simulink model "EngModelJumpRamp"  (R2013a)
settings: Solver=ode15s  StartTime=0.0  StopTime=10.0  RelTol=1e-5
values from neighbouring files (symbols this model uses):
  AFlowcontrol = AFhighc    (= 23)    [init_ele.m]
  AFn = 27*ones(engines,1)    [initHybrid.m]    (also in initMV.m; init_ele.m = 27)
  ma0 = .2*ones(engines,1)    [initHybrid.m]    (also in initMV.m; init_ele.m = 0.2)
  nr = 1    [init_ele.m]
undefined symbols (not defined in the file or in its folder): Kappa1, magnitude, pin0
undefined symbols (not defined in the file): generators
libraries: simulink x2, EngineSystemSubmodel x1
settings Model: Creator=yum  LastModifiedBy=yum
settings DebuggingCC: SolverPrmCheckMsg=none

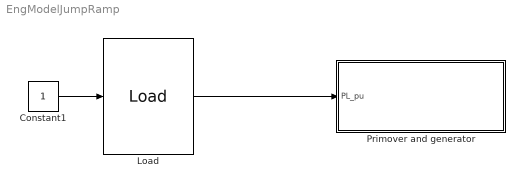
== system EngModelJumpRamp ==
  Constant1 : Constant
  Load : EngineSystemSubmodel/Load  Load_index=Load_index  Load_amp=Load_amp  Load_bias=Load_bias  Start_time=Start_time  T_load=T_load
  Primover and generator : Subsystem  mask{genset=generators(1)}
      mask prompts: genset "Genset parameters"
  wires:
  Load/1 -> Primover and generator/1(PL_pu)
  Constant1/1 -> Load/1

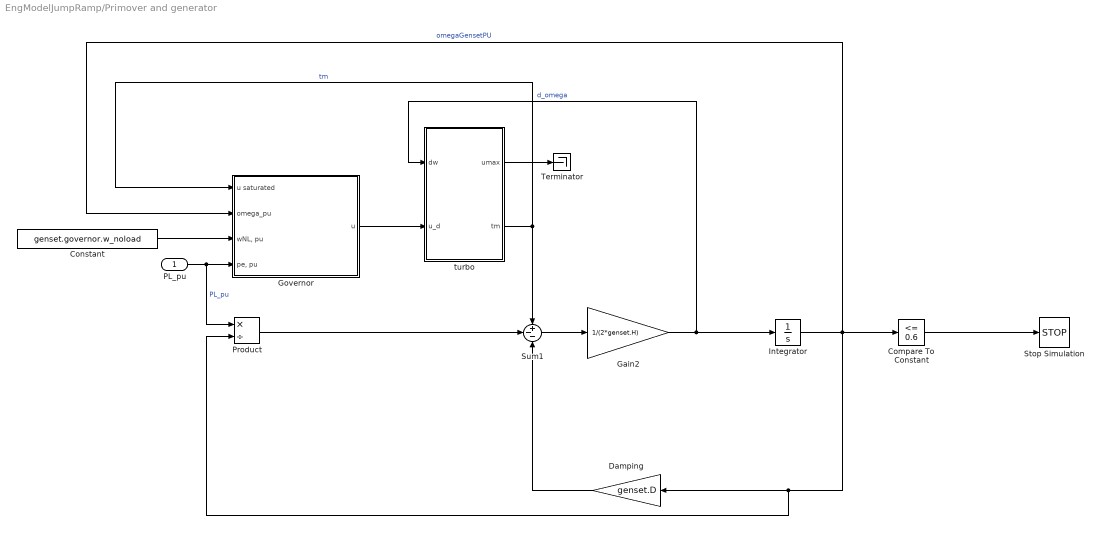
== system EngModelJumpRamp/Primover and generator ==
  PL_pu : Inport
  Compare To Constant : simulink/Logic and Bit Operations/Compare To Constant  relop=<=  const=0.6  OutDataTypeStr=boolean
  Constant : Constant  Value=genset.governor.w_noload
  Damping : Gain  Gain=genset.D
  Gain2 : Gain  Gain=1/(2*genset.H)
  Governor : Subsystem
  Integrator : Integrator  InitialCondition=genset.omega0
  Product : Product  Inputs=*/
  Stop Simulation : Stop
  Sum1 : Sum  Inputs=+--
  Terminator : Terminator
  turbo : Subsystem
  wires:
  Governor/1(u) -> turbo/2(u_d)
  turbo/2(tm) -> Sum1/1, Governor/1(u saturated)  "tm"
  Sum1/1 -> Gain2/1
  Gain2/1 -> turbo/1(dw), Integrator/1  "d_omega"
  Product/1 -> Sum1/2
  Damping/1 -> Sum1/3
  Constant/1 -> Governor/3("wNL, pu")
  PL_pu/1 -> Product/1, Governor/4("pe, pu")  "PL_pu"
  Integrator/1 -> Compare To Constant/1, Damping/1, Product/2, Governor/2(omega_pu)  "omegaGensetPU"
  Compare To Constant/1 -> Stop Simulation/1
  turbo/1(umax) -> Terminator/1

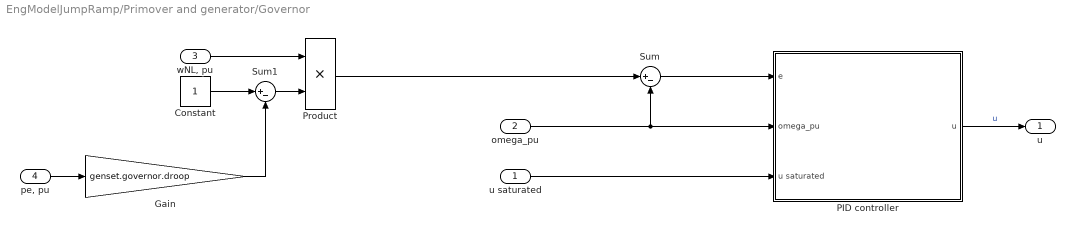
== system EngModelJumpRamp/Primover and generator/Governor ==
  u saturated : Inport
  omega_pu : Inport  Port=2
  "wNL, pu" : Inport  Port=3
  "pe, pu" : Inport  Port=4
  Constant : Constant
  Gain : Gain  Gain=genset.governor.droop
  PID controller : Subsystem
  Product : Product  RndMeth=Zero
  Sum : Sum  Inputs=|+-
  Sum1 : Sum  Inputs=|+-
  u : Outport
  wires:
  PID controller/1(u) -> u/1  "u"
  Gain/1 -> Sum1/2
  Sum/1 -> PID controller/1(e)
  Product/1 -> Sum/1
  "wNL, pu"/1 -> Product/1
  Constant/1 -> Sum1/1
  Sum1/1 -> Product/2
  u saturated/1 -> PID controller/3(u saturated)
  "pe, pu"/1 -> Gain/1
  omega_pu/1 -> Sum/2, PID controller/2(omega_pu)

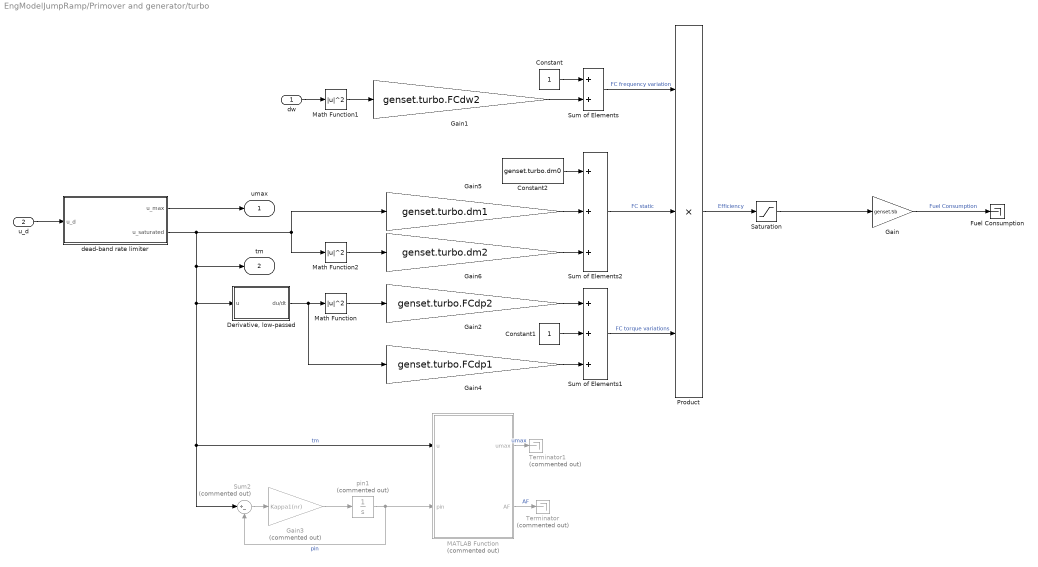
== system EngModelJumpRamp/Primover and generator/turbo ==
  dw : Inport
  u_d : Inport  Port=2
  Constant : Constant
  Constant1 : Constant
  Constant2 : Constant  Value=genset.turbo.dm0
  "Derivative, low-passed" : Subsystem
      settings: MinAlgLoopOccurrences=on
  Fuel Consumption : Terminator
  Gain : Gain  Gain=genset.Sb
  Gain1 : Gain  Gain=genset.turbo.FCdw2
  Gain2 : Gain  Gain=genset.turbo.FCdp2
  Gain3 : Gain  Commented=on  Gain=Kappa1(nr)
  Gain4 : Gain  Gain=genset.turbo.FCdp1
  Gain5 : Gain  Gain=genset.turbo.dm1
  Gain6 : Gain  Gain=genset.turbo.dm2
  MATLAB Function : MATLAB Function  Commented=on  TreatAsAtomicUnit=on
  Math Function : Math  Operator=magnitude^2  SaturateOnIntegerOverflow=on
  Math Function1 : Math  Operator=magnitude^2  SaturateOnIntegerOverflow=on
  Math Function2 : Math  Operator=magnitude^2  SaturateOnIntegerOverflow=on
  Product : Product  Inputs=3  RndMeth=Zero
  Saturation : Saturate  UpperLimit=genset.turbo.FCmax  LowerLimit=0
  Sum of Elements : Sum
  Sum of Elements1 : Sum  Inputs=+++
  Sum of Elements2 : Sum  Inputs=+++
  Sum2 : Sum  Commented=on  Inputs=|+-
  Terminator : Terminator  Commented=on
  Terminator1 : Terminator  Commented=on
  dead-band rate limiter : Subsystem  mask(Rate limiter for diesel engines){umax=genset.u_max, umin=genset.u_min}
      mask prompts: umax "Static maximum torque"; umin "Static minimum torque"
      mask help:
      | Allows the input to change within a delta limit, however if the input
      | changes more than this range will the input be saturated by a rate limiter.
  pin1 : Integrator  Commented=on  InitialCondition=pin0(nr)
  umax : Outport
  tm : Outport  Port=2
  wires:
  Gain/1 -> Fuel Consumption/1  "Fuel Consumption"
  Saturation/1 -> Gain/1
  Product/1 -> Saturation/1  "Efficiency"
  Sum of Elements/1 -> Product/1  "FC frequency variation"
  Sum of Elements2/1 -> Product/2  "FC static"
  Sum of Elements1/1 -> Product/3  "FC torque variations"
  Math Function2/1 -> Gain6/1
  Constant2/1 -> Sum of Elements2/1
  Gain5/1 -> Sum of Elements2/2
  Gain6/1 -> Sum of Elements2/3
  Constant1/1 -> Sum of Elements1/2
  Gain4/1 -> Sum of Elements1/3
  Gain2/1 -> Sum of Elements1/1
  Constant/1 -> Sum of Elements/1
  Gain1/1 -> Sum of Elements/2
  Math Function/1 -> Gain2/1
  Math Function1/1 -> Gain1/1
  "Derivative, low-passed"/1(du/dt) -> Math Function/1, Gain4/1
  pin1/1 -> MATLAB Function/2(pin), Sum2/2  "pin"
  Sum2/1 -> Gain3/1
  Gain3/1 -> pin1/1
  dead-band rate limiter/2(u_saturated) -> tm/1, Sum2/1, MATLAB Function/1(u), "Derivative, low-passed"/1(u), Gain5/1, Math Function2/1  "tm"
  u_d/1 -> dead-band rate limiter/1(u_d)
  MATLAB Function/2(AF) -> Terminator/1  "AF"
  dw/1 -> Math Function1/1
  MATLAB Function/1(umax) -> Terminator1/1  "umax"
  dead-band rate limiter/1(u_max) -> umax/1

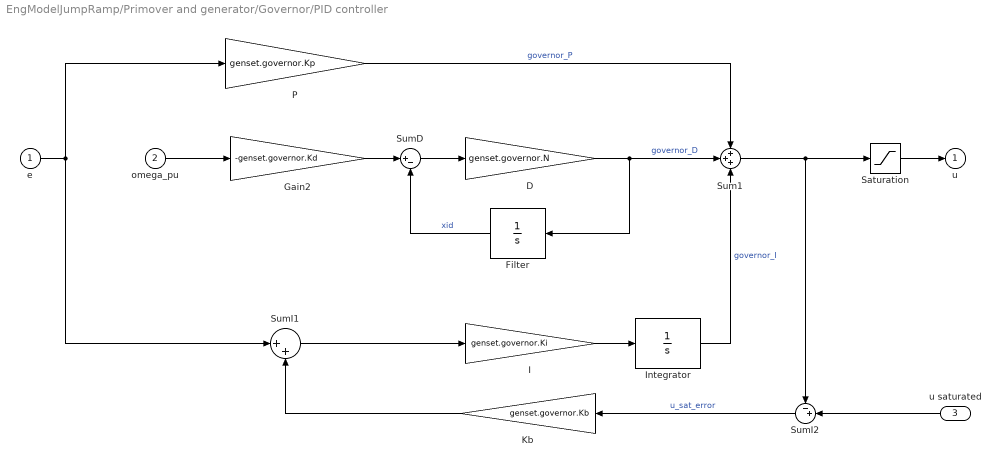
== system EngModelJumpRamp/Primover and generator/Governor/PID controller ==
  e : Inport  PortDimensions=1
  omega_pu : Inport  Port=2  PortDimensions=1
  u saturated : Inport  Port=3  PortDimensions=1
  D : Gain  DisableCoverage=on  Gain=genset.governor.N
  Filter : Integrator  DisableCoverage=on  InitialCondition=-genset.omega0*genset.governor.Kd
  Gain2 : Gain  Gain=-genset.governor.Kd
  I : Gain  Gain=genset.governor.Ki
  Integrator : Integrator  DisableCoverage=on  InitialCondition=genset.u0
  Kb : Gain  DisableCoverage=on  Gain=genset.governor.Kb  ParamDataTypeStr=Inherit: Inherit from 'Gain'
  P : Gain  Gain=genset.governor.Kp
  Saturation : Saturate  UpperLimit=genset.u_max  LowerLimit=genset.u_min  LinearizeAsGain=off  OutMin=genset.u_min  OutMax=genset.u_max  OutDataTypeStr=Inherit: Inherit via back propagation
  Sum1 : Sum  Inputs=+++
  SumD : Sum  DisableCoverage=on  Inputs=|+-
  SumI1 : Sum  DisableCoverage=on  Inputs=|++
  SumI2 : Sum  DisableCoverage=on  Inputs=-+|
  u : Outport  PortDimensions=1  InitialOutput=0
  wires:
  Integrator/1 -> Sum1/3  "governor_I"
  D/1 -> Sum1/2, Filter/1  "governor_D"
  omega_pu/1 -> Gain2/1
  e/1 -> P/1, SumI1/1
  P/1 -> Sum1/1  "governor_P"
  Saturation/1 -> u/1
  Filter/1 -> SumD/2  "xid"
  SumD/1 -> D/1
  Gain2/1 -> SumD/1
  Sum1/1 -> Saturation/1, SumI2/1
  SumI2/1 -> Kb/1  "u_sat_error"
  Kb/1 -> SumI1/2
  u saturated/1 -> SumI2/2
  SumI1/1 -> I/1
  I/1 -> Integrator/1

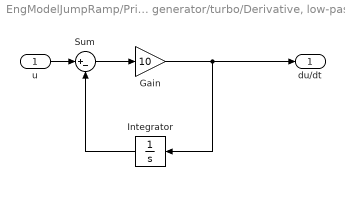
== system EngModelJumpRamp/Primover and generator/turbo/Derivative, low-passed ==
  u : Inport
  Gain : Gain  Gain=10
  Integrator : Integrator  InitialCondition=genset.u0
  Sum : Sum  Inputs=|+-
  du/dt : Outport
  wires:
  Sum/1 -> Gain/1
  Integrator/1 -> Sum/2
  Gain/1 -> du/dt/1, Integrator/1
  u/1 -> Sum/1

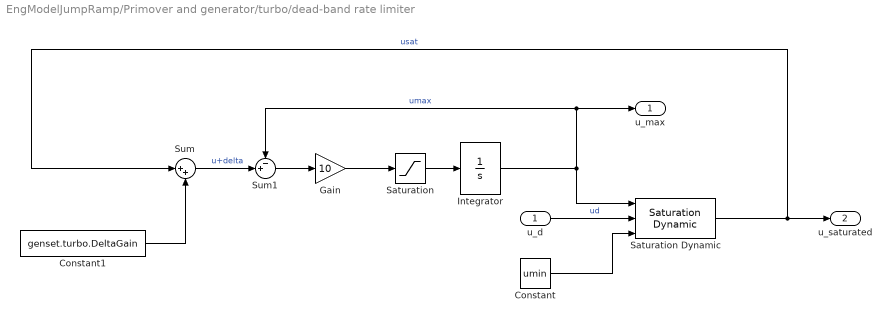
== system EngModelJumpRamp/Primover and generator/turbo/dead-band rate limiter ==
  u_d : Inport
  Constant : Constant  Value=umin
  Constant1 : Constant  Value=genset.turbo.DeltaGain
  Gain : Gain  Gain=10
  Integrator : Integrator  InitialCondition=umax  LimitOutput=on  UpperSaturationLimit=umax  LowerSaturationLimit=umin
  Saturation : Saturate  UpperLimit=genset.turbo.rateSatMax  LowerLimit=-.2
  Saturation Dynamic : simulink/Discontinuities/Saturation Dynamic  OutMin=[]  OutMax=[]  OutDataTypeStr=Inherit: Same as second input  OutDataType=fixdt(1, 16)  OutScaling=2^-10  DoSatur=off
  Sum : Sum  Inputs=|++
  Sum1 : Sum  Inputs=-+|
  u_max : Outport
  u_saturated : Outport  Port=2
  wires:
  Gain/1 -> Saturation/1
  Sum1/1 -> Gain/1
  Sum/1 -> Sum1/2  "u+delta"
  Constant/1 -> Saturation Dynamic/3
  u_d/1 -> Saturation Dynamic/2  "ud"
  Integrator/1 -> u_max/1, Sum1/1, Saturation Dynamic/1  "umax"
  Saturation/1 -> Integrator/1
  Saturation Dynamic/1 -> Sum/1, u_saturated/1  "usat"
  Constant1/1 -> Sum/2

== matlab function EngModelJumpRamp/Primover and generator/turbo/MATLAB Function ==
  data: umax output; AFn parameter; ma0 parameter; AFlowcontrol parameter; u input; pin input; AF output; nr parameter
function [umax,AF] = AF(AFn,ma0,AFlowcontrol,u,pin,nr)
umax = (ma0(nr)+(1-ma0(nr))*pin)/AFlowcontrol(nr)*AFn(nr);
AF = (ma0(nr)+(1-ma0(nr))*pin)/u*AFn(nr);
